simulink model "Vorlage_Anlagenteil_Pruefen_Gruppen12"  (R2023a)
settings: Solver=ode3  StartTime=0.0  StopTime=50  FixedStep=0.01  RelTol=1e-3
StopFcn:
  | clear con
model workspace (MAT data in the model file):
  A = Simulink.Signal
  A.DataType = 'auto'
  A.Dimensions = 1
  A.DimensionsMode = 'auto'
  A.Complexity = 'auto'
  A.SampleTime = -1
  A.SamplingMode = 'auto'
undefined symbols (not defined in the file): sigbuilder_block
libraries: simulink x11, simulink_extras x6, aerolibanimutils x1
(part 1 of 2)
settings Model: Creator=Jan  LastModifiedBy=ASUS
settings SolverCC: AlgebraicLoopSolver=TrustRegion
settings DataIOCC: ReturnWorkspaceOutputs=off
settings DebuggingCC: UnconnectedInputMsg=warning  UnconnectedOutputMsg=warning  UnconnectedLineMsg=warning  ArithmeticOperatorsInVariantConditions=warning
settings ModelReferenceCC: EnableRefExpFcnMdlSchedulingChecks=on
settings SFSimCC: SimUseLocalCustomCode=off  CustomCodeUndefinedFunction=UseInterfaceOnly
settings RTWCC: RTWUseLocalCustomCode=off  DLArmComputeVersion=19.05
settings CodeAppCC: StateflowObjectComments=on
settings SimscapeCC: SimscapeNormalizeSystem=off

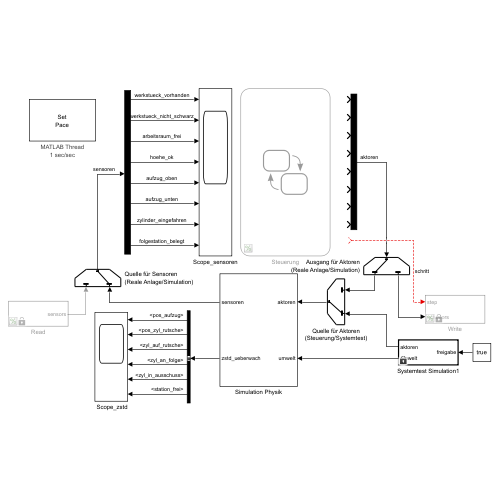
[thumbnail: Simulink's stored preview of the top-level diagram]
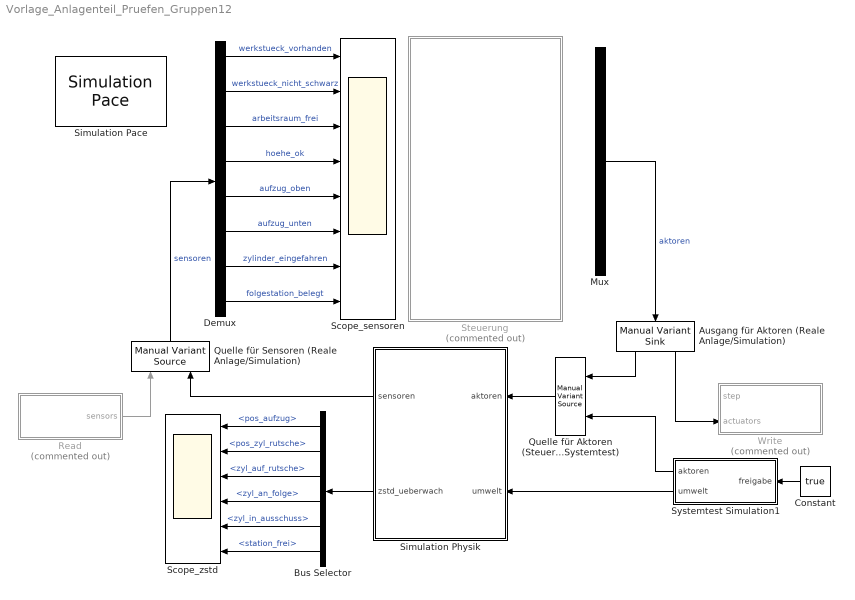
== system Vorlage_Anlagenteil_Pruefen_Gruppen12 ==
  " Scope_zstd" : Scope  NumInputPorts=6
  Ausgang für Aktoren (Reale Anlage/Simulation) : simulink/Signal Routing/Manual Variant Sink  NumChoices=2  LabelModeActiveChoice=V_1
  Bus Selector : BusSelector  OutputSignals=pos_aufzug,pos_zyl_rutsche,zyl_auf_rutsche,zyl_an_folge,zyl_in_ausschuss,station_frei
  Constant : Constant  Value=true
  Demux : Demux  Outputs=8
  Mux : Mux  Inputs=8
  Quelle für Aktoren (Steuerung/Systemtest) : simulink/Signal Routing/Manual Variant Source  NumChoices=2  LabelModeActiveChoice=V_2
  Quelle für Sensoren (Reale Anlage/Simulation) : simulink/Signal Routing/Manual Variant Source  NumChoices=2  LabelModeActiveChoice=V_2
  Read : Subsystem  Commented=on
  Scope_sensoren : Scope  NumInputPorts=8
  Simulation Pace : aerolibanimutils/Simulation Pace  SimulationPace=1  SleepMode=MATLAB Thread  OutputPaceError=off  SampleTime=-1
  Simulation Physik : Subsystem
  Steuerung : Stateflow chart  Commented=on  TreatAsAtomicUnit=on
  Systemtest Simulation1 : Subsystem  TreatAsAtomicUnit=on
  Write : Subsystem  Commented=on
  wires:
  Quelle für Sensoren (Reale Anlage/Simulation)/1 -> Demux/1  "sensoren"
  Read/1(sensors) -> Quelle für Sensoren (Reale Anlage/Simulation)/1
  Mux/1 -> Ausgang für Aktoren (Reale Anlage/Simulation)/1  "aktoren"
  Simulation Physik/1(sensoren) -> Quelle für Sensoren (Reale Anlage/Simulation)/2
  Ausgang für Aktoren (Reale Anlage/Simulation)/2 -> Write/2(actuators)
  Ausgang für Aktoren (Reale Anlage/Simulation)/1 -> Quelle für Aktoren (Steuerung/Systemtest)/1
  Quelle für Aktoren (Steuerung/Systemtest)/1 -> Simulation Physik/1(aktoren)
  Systemtest Simulation1/1(aktoren) -> Quelle für Aktoren (Steuerung/Systemtest)/2
  Systemtest Simulation1/2(umwelt) -> Simulation Physik/2(umwelt)
  Simulation Physik/2(zstd_ueberwach) -> Bus Selector/1
  Bus Selector/1 -> " Scope_zstd"/1  "<pos_aufzug>"
  Bus Selector/2 -> " Scope_zstd"/2  "<pos_zyl_rutsche>"
  Bus Selector/3 -> " Scope_zstd"/3  "<zyl_auf_rutsche>"
  Bus Selector/4 -> " Scope_zstd"/4  "<zyl_an_folge>"
  Bus Selector/5 -> " Scope_zstd"/5  "<zyl_in_ausschuss>"
  Bus Selector/6 -> " Scope_zstd"/6  "<station_frei>"
  Demux/1 -> Scope_sensoren/1  "werkstueck_vorhanden"
  Demux/2 -> Scope_sensoren/2  "werkstueck_nicht_schwarz"
  Demux/3 -> Scope_sensoren/3  "arbeitsraum_frei"
  Demux/4 -> Scope_sensoren/4  "hoehe_ok"
  Demux/5 -> Scope_sensoren/5  "aufzug_oben"
  Demux/6 -> Scope_sensoren/6  "aufzug_unten"
  Demux/7 -> Scope_sensoren/7  "zylinder_eingefahren"
  Demux/8 -> Scope_sensoren/8  "folgestation_belegt"
  ? -> Write/1(step)  "schritt"
  Constant/1 -> Systemtest Simulation1/1(freigabe)

== system Vorlage_Anlagenteil_Pruefen_Gruppen12/Read ==
  Read : MATLAB Function  TreatAsAtomicUnit=on
  sensors : Outport  VectorParamsAs1DForOutWhenUnconnected=off
  wires:
  Read/1(senarr) -> sensors/1

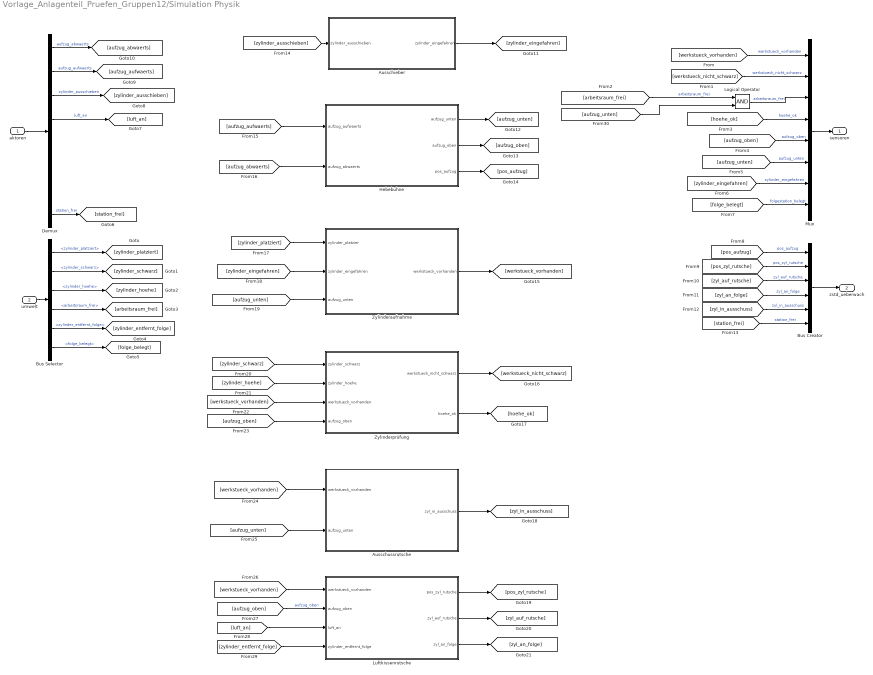
== system Vorlage_Anlagenteil_Pruefen_Gruppen12/Simulation Physik ==
  aktoren : Inport
  umwelt : Inport  Port=2
  Ausschieber : Subsystem
  Ausschussrutsche : Subsystem  TreatAsAtomicUnit=on
  Bus Creator : BusCreator  Inputs=6
  Bus Selector : BusSelector  OutputSignals=zylinder_platziert,zylinder_schwarz,zylinder_hoehe,arbeitsraum_frei,zylinder_entfernt_folge,folge_belegt
  Demux : Demux  Outputs=8
  "Hebebühne " : Subsystem
  Logical Operator : Logic  AllPortsSameDT=off  OutDataTypeStr=boolean
  Luftkissenrutsche : Subsystem
  Mux : Mux  Inputs=8
  Zylinderaufnahme : Subsystem
  Zylinderprüfung : Subsystem
  sensoren : Outport  VectorParamsAs1DForOutWhenUnconnected=off
  zstd_ueberwach : Outport  Port=2  VectorParamsAs1DForOutWhenUnconnected=off
  wires:
  aktoren/1 -> Demux/1
  Mux/1 -> sensoren/1
  Demux/1 -> [aufzug_abwaerts]  "aufzug_abwaerts"
  [folge_belegt] -> Mux/8  "folgestation_belegt"
  Demux/2 -> [aufzug_aufwaerts]  "aufzug_aufwaerts"
  Demux/3 -> [zylinder_ausschieben]  "zylinder_ausschieben"
  [werkstueck_vorhanden] -> Mux/1  "werkstueck_vorhanden"
  [hoehe_ok] -> Mux/4  "hoehe_ok"
  [werkstueck_nicht_schwarz] -> Mux/2  "werkstueck_nicht_schwarz"
  umwelt/1 -> Bus Selector/1
  Bus Selector/1 -> [zylinder_platziert]  "<zylinder_platziert>"
  Bus Selector/2 -> [zylinder_schwarz]  "<zylinder_schwarz>"
  Bus Selector/4 -> [arbeitsraum_frei]  "<arbeitsraum_frei>"
  Bus Selector/5 -> [zylinder_entfernt_folge]  "<zylinder_entfernt_folge>"
  Bus Selector/6 -> [folge_belegt]  "<folge_belegt>"
  [pos_aufzug] -> Bus Creator/1  "pos_aufzug"
  Bus Creator/1 -> zstd_ueberwach/1
  [pos_zyl_rutsche] -> Bus Creator/2  "pos_zyl_rutsche"
  [zyl_auf_rutsche] -> Bus Creator/3  "zyl_auf_rutsche"
  [zyl_an_folge] -> Bus Creator/4  "zyl_an_folge"
  [zyl_in_ausschuss] -> Bus Creator/5  "zyl_in_ausschuss"
  [aufzug_unten] -> Mux/6  "aufzug_unten"
  [zylinder_eingefahren] -> Mux/7  "zylinder_eingefahren"
  [aufzug_oben] -> Mux/5  "aufzug_oben"
  Bus Selector/3 -> [zylinder_hoehe]  "<zylinder_hoehe>"
  Demux/8 -> [station_frei]  "station_frei"
  [station_frei] -> Bus Creator/6  "station_frei"
  Demux/4 -> [luft_an]  "luft_an"
  [zylinder_ausschieben] -> Ausschieber/1(zylinder_ausschieben)
  Ausschieber/1(zylinder_eingefahren) -> [zylinder_eingefahren]
  [aufzug_aufwaerts] -> "Hebebühne "/1(aufzug_aufwaerts)
  [aufzug_abwaerts] -> "Hebebühne "/2(aufzug_abwaerts)
  "Hebebühne "/1(aufzug_unten) -> [aufzug_unten]
  "Hebebühne "/2(aufzug_oben) -> [aufzug_oben]
  "Hebebühne "/3(pos_aufzug) -> [pos_aufzug]
  [aufzug_unten] -> Zylinderaufnahme/3(aufzug_unten)
  [zylinder_eingefahren] -> Zylinderaufnahme/2(zylinder_eingefahren)
  [zylinder_platziert] -> Zylinderaufnahme/1(zylinder_platzier)
  Zylinderaufnahme/1(werkstueck_vorhanden) -> [werkstueck_vorhanden]
  [zylinder_schwarz] -> Zylinderprüfung/1(zylinder_schwarz)
  [zylinder_hoehe] -> Zylinderprüfung/2(zylinder_hoehe)
  [werkstueck_vorhanden] -> Zylinderprüfung/3(werkstueck_vorhanden)
  [aufzug_oben] -> Zylinderprüfung/4("aufzug_oben ")
  Zylinderprüfung/1(werkstueck_nicht_schwarz) -> [werkstueck_nicht_schwarz]
  Zylinderprüfung/2(hoehe_ok) -> [hoehe_ok]
  [aufzug_unten] -> Ausschussrutsche/2("aufzug_unten ")
  [werkstueck_vorhanden] -> Ausschussrutsche/1(werkstueck_vorhanden)
  Ausschussrutsche/1(zyl_in_ausschuss) -> [zyl_in_ausschuss]
  Luftkissenrutsche/1(pos_zyl_rutsche) -> [pos_zyl_rutsche]
  Luftkissenrutsche/3(zyl_an_folge) -> [zyl_an_folge]
  Luftkissenrutsche/2(zyl_auf_rutsche) -> [zyl_auf_rutsche]
  [werkstueck_vorhanden] -> Luftkissenrutsche/1("werkstueck_vorhanden ")
  [aufzug_oben] -> Luftkissenrutsche/2("aufzug_oben ")  "aufzug_oben"
  [luft_an] -> Luftkissenrutsche/3(luft_an)
  [zylinder_entfernt_folge] -> Luftkissenrutsche/4(zylinder_entfernt_folge)
  [arbeitsraum_frei] -> Logical Operator/1  "arbeitsraum_frei"
  Logical Operator/1 -> Mux/3  "arbeitsraum_frei"
  [aufzug_unten] -> Logical Operator/2

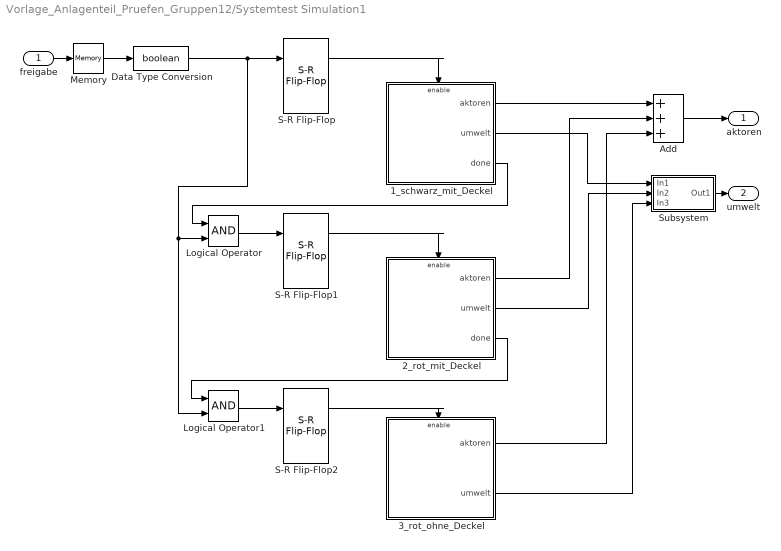
== system Vorlage_Anlagenteil_Pruefen_Gruppen12/Systemtest Simulation1 ==
  freigabe : Inport
  1_schwarz_mit_Deckel : Subsystem
  2_rot_mit_Deckel : Subsystem
  3_rot_ohne_Deckel : Subsystem
  Add : Sum  Inputs=+++
  Data Type Conversion : DataTypeConversion  OutDataTypeStr=boolean  SaturateOnIntegerOverflow=off  RndMeth=Floor
  Logical Operator : Logic  AllPortsSameDT=off  OutDataTypeStr=boolean
  Logical Operator1 : Logic  AllPortsSameDT=off  OutDataTypeStr=boolean
  Memory : Memory
  S-R Flip-Flop : simulink_extras/Flip Flops/S-R Flip-Flop  initial_condition=0
  S-R Flip-Flop1 : simulink_extras/Flip Flops/S-R Flip-Flop  initial_condition=0
  S-R Flip-Flop2 : simulink_extras/Flip Flops/S-R Flip-Flop  initial_condition=0
  Subsystem : Subsystem
  aktoren : Outport  VectorParamsAs1DForOutWhenUnconnected=off
  umwelt : Outport  Port=2  VectorParamsAs1DForOutWhenUnconnected=off
  wires:
  freigabe/1 -> Memory/1
  S-R Flip-Flop/1 -> 1_schwarz_mit_Deckel/Enable
  Logical Operator/1 -> S-R Flip-Flop1/1
  1_schwarz_mit_Deckel/3(done) -> Logical Operator/1
  S-R Flip-Flop1/1 -> 2_rot_mit_Deckel/Enable
  Logical Operator1/1 -> S-R Flip-Flop2/1
  2_rot_mit_Deckel/3(done) -> Logical Operator1/1
  S-R Flip-Flop2/1 -> 3_rot_ohne_Deckel/Enable
  1_schwarz_mit_Deckel/1(aktoren) -> Add/1
  2_rot_mit_Deckel/1(aktoren) -> Add/2
  Add/1 -> aktoren/1
  3_rot_ohne_Deckel/1(aktoren) -> Add/3
  Subsystem/1(Out1) -> umwelt/1
  1_schwarz_mit_Deckel/2(umwelt) -> Subsystem/1(In1)
  2_rot_mit_Deckel/2(umwelt) -> Subsystem/2(In2)
  3_rot_ohne_Deckel/2(umwelt) -> Subsystem/3(In3)
  Data Type Conversion/1 -> Logical Operator1/2, Logical Operator/2, S-R Flip-Flop/1
  Memory/1 -> Data Type Conversion/1

== system Vorlage_Anlagenteil_Pruefen_Gruppen12/Write ==
  step : Inport
  actuators : Inport  Port=2
  Data Type Conversion : DataTypeConversion  OutDataTypeStr=boolean  SaturateOnIntegerOverflow=off  RndMeth=Floor
  Write1 : MATLAB Function  TreatAsAtomicUnit=on
  wires:
  step/1 -> Write1/1(step)
  Data Type Conversion/1 -> Write1/2(actuators)
  actuators/1 -> Data Type Conversion/1

== system Vorlage_Anlagenteil_Pruefen_Gruppen12/Simulation Physik/Ausschieber ==
  zylinder_ausschieben : Inport
  " " : Logic  Operator=NOT  AllPortsSameDT=off  OutDataTypeStr=boolean
  "  " : Delay  DelayLength=50
  Scope : Scope  NumInputPorts=2
  zylinder_eingefahren : Outport
  wires:
  zylinder_ausschieben/1 -> Scope/2, " "/1  "zylinder_ausschieben"
  " "/1 -> "  "/1
  "  "/1 -> Scope/1, zylinder_eingefahren/1  "zylinder_eingefahren"

== system Vorlage_Anlagenteil_Pruefen_Gruppen12/Simulation Physik/Ausschussrutsche ==
  werkstueck_vorhanden : Inport
  "aufzug_unten " : Inport  Port=2
  AND : Logic  IconShape=distinctive  AllPortsSameDT=off  OutDataTypeStr=boolean
  Detect Fall Nonpositive : simulink/Logic and Bit Operations/Detect Fall Nonpositive  vinit=0  OutDataTypeStr=boolean
  Scope : Scope  NumInputPorts=3
  Triggered Subsystem : Subsystem  TreatAsAtomicUnit=on
  zyl_in_ausschuss : Outport
  wires:
  werkstueck_vorhanden/1 -> Scope/1, Detect Fall Nonpositive/1  "werkstueck_vorhanden"
  Detect Fall Nonpositive/1 -> AND/1
  "aufzug_unten "/1 -> Scope/2, AND/2  "aufzug_unten"
  AND/1 -> Triggered Subsystem/Trigger
  Triggered Subsystem/1(zyl_in_ausschuss) -> Scope/3, zyl_in_ausschuss/1  "zyl_in_ausschuss"

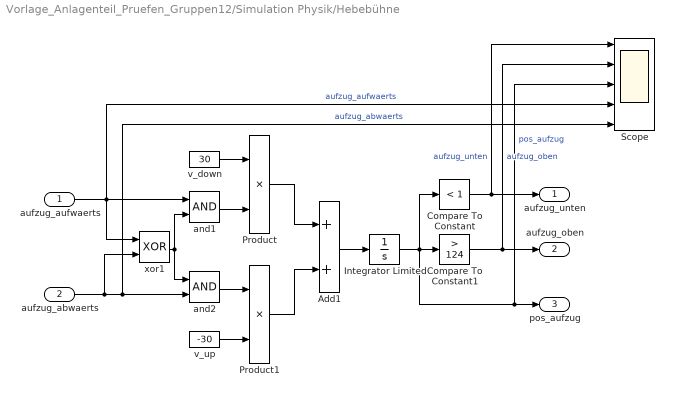
== system Vorlage_Anlagenteil_Pruefen_Gruppen12/Simulation Physik/Hebebühne  ==
  aufzug_aufwaerts : Inport
  aufzug_abwaerts : Inport  Port=2
  Add1 : Sum
  Compare To Constant : simulink/Logic and Bit Operations/Compare To Constant  relop=<  const=1  OutDataTypeStr=boolean
  Compare To Constant1 : simulink/Logic and Bit Operations/Compare To Constant  relop=>  const=124  OutDataTypeStr=boolean
  Integrator Limited : Integrator  LimitOutput=on  UpperSaturationLimit=125  LowerSaturationLimit=0
  Product : Product
  Product1 : Product
  Scope : Scope  NumInputPorts=5
  and1 : Logic  AllPortsSameDT=off  OutDataTypeStr=boolean
  and2 : Logic  AllPortsSameDT=off  OutDataTypeStr=boolean
  v_down : Constant  Value=30
  v_up : Constant  Value=-30
  xor1 : Logic  Operator=XOR  AllPortsSameDT=off  OutDataTypeStr=boolean
  aufzug_unten : Outport
  aufzug_oben : Outport  Port=2
  pos_aufzug : Outport  Port=3
  wires:
  Compare To Constant/1 -> Scope/1, aufzug_unten/1  "aufzug_unten"
  Integrator Limited/1 -> pos_aufzug/1, Scope/3, Compare To Constant/1, Compare To Constant1/1  "pos_aufzug"
  Add1/1 -> Integrator Limited/1
  Product1/1 -> Add1/2
  Product/1 -> Add1/1
  v_up/1 -> Product1/2
  and2/1 -> Product1/1
  v_down/1 -> Product/1
  and1/1 -> Product/2
  xor1/1 -> and1/2, and2/1
  aufzug_aufwaerts/1 -> Scope/4, and1/1, xor1/1  "aufzug_aufwaerts"
  aufzug_abwaerts/1 -> Scope/5, and2/2, xor1/2  "aufzug_abwaerts"
  Compare To Constant1/1 -> aufzug_oben/1, Scope/2  "aufzug_oben"

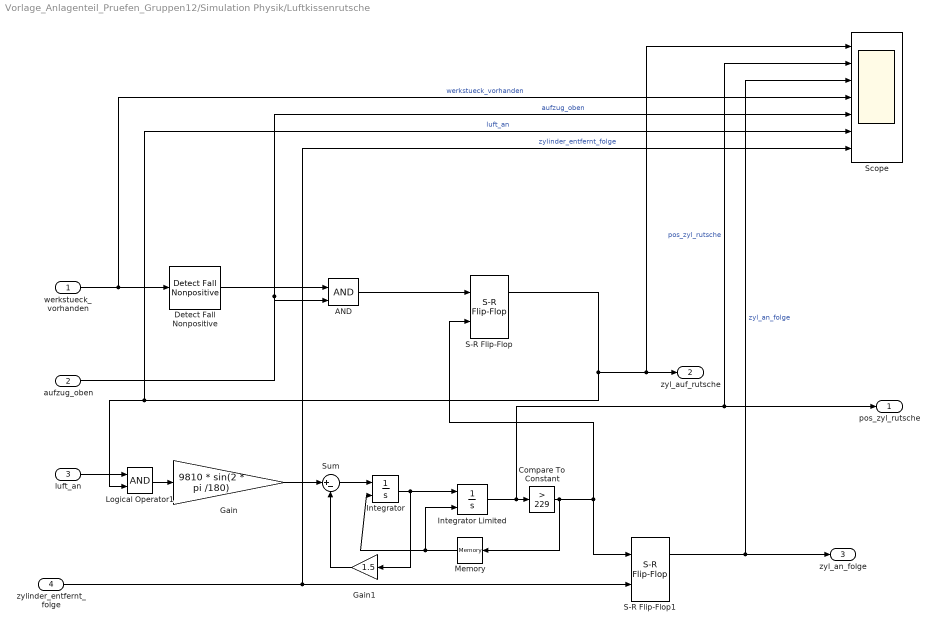
== system Vorlage_Anlagenteil_Pruefen_Gruppen12/Simulation Physik/Luftkissenrutsche ==
  "werkstueck_vorhanden " : Inport
  "aufzug_oben " : Inport  Port=2
  luft_an : Inport  Port=3
  zylinder_entfernt_folge : Inport  Port=4
  AND : Logic  IconShape=distinctive  AllPortsSameDT=off  OutDataTypeStr=boolean
  Compare To Constant : simulink/Logic and Bit Operations/Compare To Constant  relop=>  const=229  OutDataTypeStr=boolean
  Detect Fall Nonpositive : simulink/Logic and Bit Operations/Detect Fall Nonpositive  vinit=0  OutDataTypeStr=boolean
  Gain : Gain  Gain=9810 * sin(2 * pi /180)
  Gain1 : Gain  Gain=1.5
  Integrator : Integrator  ExternalReset=rising
  Integrator Limited : Integrator  ExternalReset=rising  LimitOutput=on  UpperSaturationLimit=230  LowerSaturationLimit=0
  Logical Operator1 : Logic  AllPortsSameDT=off  OutDataTypeStr=boolean
  Memory : Memory
  S-R Flip-Flop : simulink_extras/Flip Flops/S-R Flip-Flop  initial_condition=0
  S-R Flip-Flop1 : simulink_extras/Flip Flops/S-R Flip-Flop  initial_condition=0
  Scope : Scope  NumInputPorts=7
  Sum : Sum  Inputs=|+-
  pos_zyl_rutsche : Outport
  zyl_auf_rutsche : Outport  Port=2
  zyl_an_folge : Outport  Port=3
  wires:
  "werkstueck_vorhanden "/1 -> Scope/4, Detect Fall Nonpositive/1  "werkstueck_vorhanden"
  Detect Fall Nonpositive/1 -> AND/1
  "aufzug_oben "/1 -> Scope/5, AND/2  "aufzug_oben"
  zylinder_entfernt_folge/1 -> Scope/7, S-R Flip-Flop1/2  "zylinder_entfernt_folge"
  S-R Flip-Flop1/1 -> Scope/3, zyl_an_folge/1  "zyl_an_folge"
  Gain1/1 -> Sum/2
  Memory/1 -> Integrator/2, Integrator Limited/2
  Compare To Constant/1 -> S-R Flip-Flop/2, S-R Flip-Flop1/1, Memory/1
  Integrator Limited/1 -> pos_zyl_rutsche/1, Scope/2, Compare To Constant/1  "pos_zyl_rutsche"
  Integrator/1 -> Integrator Limited/1, Gain1/1
  Sum/1 -> Integrator/1
  Gain/1 -> Sum/1
  Logical Operator1/1 -> Gain/1
  luft_an/1 -> Logical Operator1/1
  S-R Flip-Flop/1 -> Scope/1, zyl_auf_rutsche/1, Logical Operator1/2, Scope/6  "luft_an"
  AND/1 -> S-R Flip-Flop/1

== system Vorlage_Anlagenteil_Pruefen_Gruppen12/Simulation Physik/Zylinderaufnahme ==
  zylinder_platzier : Inport
  zylinder_eingefahren : Inport  Port=2
  aufzug_unten : Inport  Port=3
  Detect Fall Nonpositive : simulink/Logic and Bit Operations/Detect Fall Nonpositive  vinit=0  OutDataTypeStr=boolean
  Detect Rise Positive : simulink/Logic and Bit Operations/Detect Rise Positive  vinit=0  OutDataTypeStr=boolean
  Logical Operator : Logic  Inputs=3  AllPortsSameDT=off  OutDataTypeStr=boolean
  S-R Flip-Flop : simulink_extras/Flip Flops/S-R Flip-Flop  initial_condition=0
  Scope : Scope  NumInputPorts=4
  werkstueck_vorhanden : Outport
  wires:
  zylinder_platzier/1 -> Scope/2, Detect Rise Positive/1  "zylinder_platzier"
  Detect Rise Positive/1 -> Logical Operator/1
  aufzug_unten/1 -> Scope/4, Logical Operator/3  "aufzug_unten"
  zylinder_eingefahren/1 -> Scope/3, Logical Operator/2, Detect Fall Nonpositive/1  "zylinder_eingefahren"
  Detect Fall Nonpositive/1 -> S-R Flip-Flop/2
  Logical Operator/1 -> S-R Flip-Flop/1
  S-R Flip-Flop/1 -> Scope/1, werkstueck_vorhanden/1  "werkstueck_vorhanden"

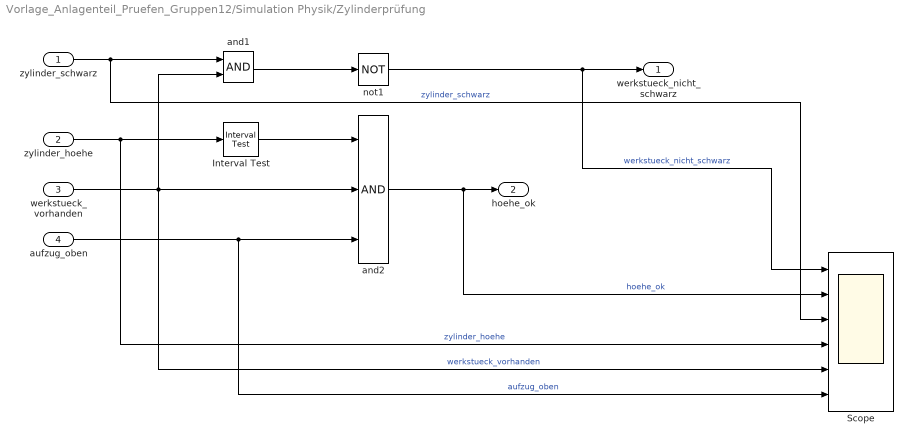
== system Vorlage_Anlagenteil_Pruefen_Gruppen12/Simulation Physik/Zylinderprüfung ==
  zylinder_schwarz : Inport
  zylinder_hoehe : Inport  Port=2
  werkstueck_vorhanden : Inport  Port=3
  "aufzug_oben " : Inport  Port=4
  Interval Test : simulink/Logic and Bit Operations/Interval Test  IntervalClosedRight=on  uplimit=26  IntervalClosedLeft=on  lowlimit=24  OutDataTypeStr=boolean
  Scope : Scope  NumInputPorts=6
  and1 : Logic  AllPortsSameDT=off  OutDataTypeStr=boolean
  and2 : Logic  Inputs=3  AllPortsSameDT=off  OutDataTypeStr=boolean
  not1 : Logic  Operator=NOT  AllPortsSameDT=off  OutDataTypeStr=boolean
  werkstueck_nicht_schwarz : Outport
  hoehe_ok : Outport  Port=2
  wires:
  zylinder_schwarz/1 -> Scope/3, and1/1  "zylinder_schwarz"
  werkstueck_vorhanden/1 -> Scope/5, and1/2, and2/2  "werkstueck_vorhanden"
  and1/1 -> not1/1
  not1/1 -> Scope/1, werkstueck_nicht_schwarz/1  "werkstueck_nicht_schwarz"
  zylinder_hoehe/1 -> Scope/4, Interval Test/1  "zylinder_hoehe"
  and2/1 -> Scope/2, hoehe_ok/1  "hoehe_ok"
  Interval Test/1 -> and2/1
  "aufzug_oben "/1 -> Scope/6, and2/3  "aufzug_oben"

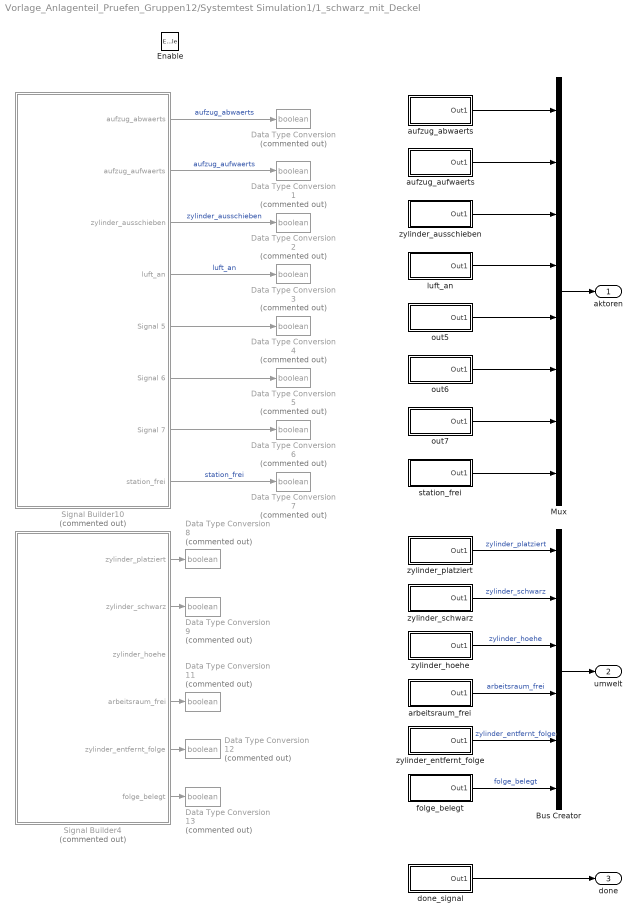
== system Vorlage_Anlagenteil_Pruefen_Gruppen12/Systemtest Simulation1/1_schwarz_mit_Deckel ==
  Enable : EnablePort
  Bus Creator : BusCreator  Inputs=6
  Data Type Conversion{,1..9,11..13} (13 alike) : DataTypeConversion  Commented=on  OutDataTypeStr=boolean  SaturateOnIntegerOverflow=off  RndMeth=Floor
  Mux : Mux  Inputs=8
  Signal Builder10 : Subsystem  Tag=STV Subsys  Commented=on  LoadFcn=sigbuilder_block('load');  StartFcn=sigbuilder_block('start');  StopFcn=sigbuilder_block('stop');  ClipboardFcn=sigbuilder_block('clipboard');  mask(Sigbuilder block){tuvar=[0:10]}
      mask help: Simulink:masks:SigbuilderBlock_MD
      mask init:
      | if ~strcmp(get_param(bdroot(gcbh),'SimulationStatus'),'stopped') tuvar = sigbuilder_block('maskInit'); end
      settings: CopyFcn=sigbuilder_block('copy');  DeleteFcn=sigbuilder_block('delete');  ModelCloseFcn=sigbuilder_block('modelClose');  PreSaveFcn=sigbuilder_block('preSave');  PauseFcn=sigbuilder_block('pause');  ContinueFcn=sigbuilder_block('continue');  NameChangeFcn=sigbuilder_block('namechange');  OpenFcn=sigbuilder_block('open',[2160 -195 1440 817.5 ]);  CloseFcn=sigbuilder_block('close');
      mask Display: plot(0, 0, 100, 100,[2, 2, 32, 32, 2], [68, 8, 8, 68, 68],[32, 2], [38, 38], [32, 19, 2],[53, 60, 44], [32, 17, 17, 2],[16, 16, 31, 31]);txt = getActiveGroup(gcbh);text(2, 100, txt,'verticalAlignment', 'top');
  Signal Builder4 : Subsystem  Tag=STV Subsys  Commented=on  LoadFcn=sigbuilder_block('load');  StartFcn=sigbuilder_block('start');  StopFcn=sigbuilder_block('stop');  ClipboardFcn=sigbuilder_block('clipboard');  mask(Sigbuilder block){tuvar=[0:10]}
      mask help: Simulink:masks:SigbuilderBlock_MD
      mask init:
      | if ~strcmp(get_param(bdroot(gcbh),'SimulationStatus'),'stopped') tuvar = sigbuilder_block('maskInit'); end
      settings: CopyFcn=sigbuilder_block('copy');  DeleteFcn=sigbuilder_block('delete');  ModelCloseFcn=sigbuilder_block('modelClose');  PreSaveFcn=sigbuilder_block('preSave');  PauseFcn=sigbuilder_block('pause');  ContinueFcn=sigbuilder_block('continue');  NameChangeFcn=sigbuilder_block('namechange');  OpenFcn=sigbuilder_block('open',[4.875 4.875 1070.25 612.75 ]);  CloseFcn=sigbuilder_block('close');
      mask Display: plot(0, 0, 100, 100,[2, 2, 32, 32, 2], [68, 8, 8, 68, 68],[32, 2], [38, 38], [32, 19, 2],[53, 60, 44], [32, 17, 17, 2],[16, 16, 31, 31]);txt = getActiveGroup(gcbh);text(2, 100, txt,'verticalAlignment', 'top');
  arbeitsraum_frei : Subsystem
  aufzug_abwaerts : Subsystem
  aufzug_aufwaerts : Subsystem
  done_signal : Subsystem
  folge_belegt : Subsystem
  luft_an : Subsystem
  out5 : Subsystem
  out6 : Subsystem
  out7 : Subsystem
  station_frei : Subsystem
  zylinder_ausschieben : Subsystem
  zylinder_entfernt_folge : Subsystem
  zylinder_hoehe : Subsystem
  zylinder_platziert : Subsystem
  zylinder_schwarz : Subsystem
  aktoren : Outport  VectorParamsAs1DForOutWhenUnconnected=off
  umwelt : Outport  Port=2  VectorParamsAs1DForOutWhenUnconnected=off
  done : Outport  Port=3  VectorParamsAs1DForOutWhenUnconnected=off
  wires:
  Bus Creator/1 -> umwelt/1
  Signal Builder4/1(zylinder_platziert) -> Data Type Conversion8/1
  Signal Builder4/2(zylinder_schwarz) -> Data Type Conversion9/1
  zylinder_hoehe/1(Out1) -> Bus Creator/3  "zylinder_hoehe"
  Signal Builder4/4(arbeitsraum_frei) -> Data Type Conversion11/1
  Signal Builder4/5(zylinder_entfernt_folge) -> Data Type Conversion12/1
  Signal Builder4/6(folge_belegt) -> Data Type Conversion13/1
  zylinder_platziert/1(Out1) -> Bus Creator/1  "zylinder_platziert"
  zylinder_schwarz/1(Out1) -> Bus Creator/2  "zylinder_schwarz"
  arbeitsraum_frei/1(Out1) -> Bus Creator/4  "arbeitsraum_frei"
  zylinder_entfernt_folge/1(Out1) -> Bus Creator/5  "zylinder_entfernt_folge"
  folge_belegt/1(Out1) -> Bus Creator/6  "folge_belegt"
  Mux/1 -> aktoren/1
  Signal Builder10/1(aufzug_abwaerts) -> Data Type Conversion/1  "aufzug_abwaerts"
  Signal Builder10/2(aufzug_aufwaerts) -> Data Type Conversion1/1  "aufzug_aufwaerts"
  Signal Builder10/3(zylinder_ausschieben) -> Data Type Conversion2/1  "zylinder_ausschieben"
  Signal Builder10/4(luft_an) -> Data Type Conversion3/1  "luft_an"
  Signal Builder10/8(station_frei) -> Data Type Conversion7/1  "station_frei"
  Signal Builder10/5(Signal 5) -> Data Type Conversion4/1
  Signal Builder10/6(Signal 6) -> Data Type Conversion5/1
  Signal Builder10/7(Signal 7) -> Data Type Conversion6/1
  aufzug_abwaerts/1(Out1) -> Mux/1
  aufzug_aufwaerts/1(Out1) -> Mux/2
  zylinder_ausschieben/1(Out1) -> Mux/3
  luft_an/1(Out1) -> Mux/4
  out5/1(Out1) -> Mux/5
  out6/1(Out1) -> Mux/6
  out7/1(Out1) -> Mux/7
  station_frei/1(Out1) -> Mux/8
  done_signal/1(Out1) -> done/1

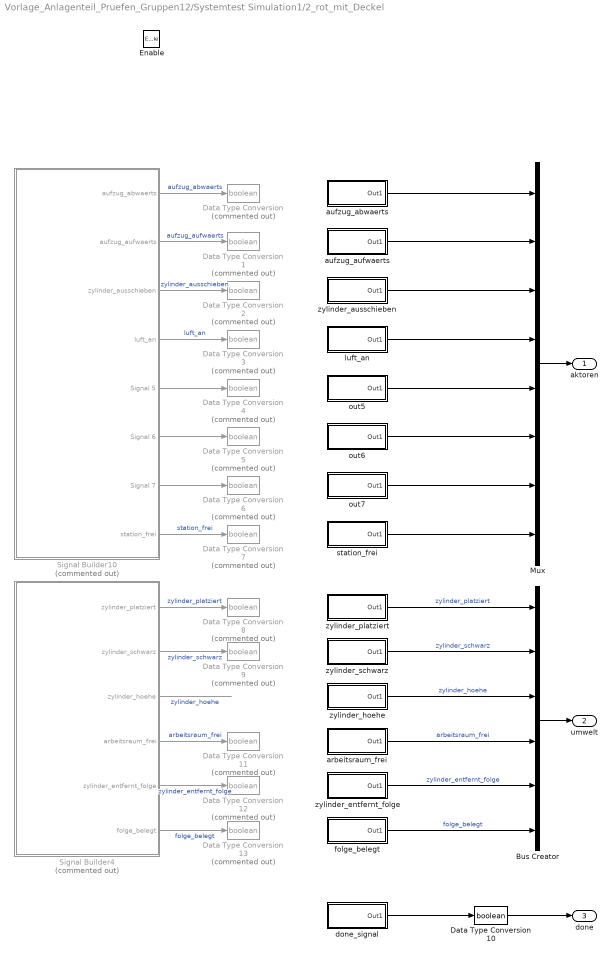
== system Vorlage_Anlagenteil_Pruefen_Gruppen12/Systemtest Simulation1/2_rot_mit_Deckel ==
  Enable : EnablePort
  Bus Creator : BusCreator  Inputs=6
  Data Type Conversion{,1..9,11..13} (13 alike) : DataTypeConversion  Commented=on  OutDataTypeStr=boolean  SaturateOnIntegerOverflow=off  RndMeth=Floor
  Data Type Conversion10 : DataTypeConversion  OutDataTypeStr=boolean  SaturateOnIntegerOverflow=off  RndMeth=Floor
  Mux : Mux  Inputs=8
  Signal Builder10 : Subsystem  Tag=STV Subsys  Commented=on  LoadFcn=sigbuilder_block('load');  StartFcn=sigbuilder_block('start');  StopFcn=sigbuilder_block('stop');  ClipboardFcn=sigbuilder_block('clipboard');  mask(Sigbuilder block){tuvar=[0:10]}
      mask help: Simulink:masks:SigbuilderBlock_MD
      mask init:
      | if ~strcmp(get_param(bdroot(gcbh),'SimulationStatus'),'stopped') tuvar = sigbuilder_block('maskInit'); end
      settings: CopyFcn=sigbuilder_block('copy');  DeleteFcn=sigbuilder_block('delete');  ModelCloseFcn=sigbuilder_block('modelClose');  PreSaveFcn=sigbuilder_block('preSave');  PauseFcn=sigbuilder_block('pause');  ContinueFcn=sigbuilder_block('continue');  NameChangeFcn=sigbuilder_block('namechange');  OpenFcn=sigbuilder_block('open',[4.875 4.875 1070.25 612.75 ]);  CloseFcn=sigbuilder_block('close');
      mask Display: plot(0, 0, 100, 100,[2, 2, 32, 32, 2], [68, 8, 8, 68, 68],[32, 2], [38, 38], [32, 19, 2],[53, 60, 44], [32, 17, 17, 2],[16, 16, 31, 31]);txt = getActiveGroup(gcbh);text(2, 100, txt,'verticalAlignment', 'top');
  Signal Builder4 : Subsystem  Tag=STV Subsys  Commented=on  LoadFcn=sigbuilder_block('load');  StartFcn=sigbuilder_block('start');  StopFcn=sigbuilder_block('stop');  ClipboardFcn=sigbuilder_block('clipboard');  mask(Sigbuilder block){tuvar=[0:10]}
      mask help: Simulink:masks:SigbuilderBlock_MD
      mask init:
      | if ~strcmp(get_param(bdroot(gcbh),'SimulationStatus'),'stopped') tuvar = sigbuilder_block('maskInit'); end
      settings: CopyFcn=sigbuilder_block('copy');  DeleteFcn=sigbuilder_block('delete');  ModelCloseFcn=sigbuilder_block('modelClose');  PreSaveFcn=sigbuilder_block('preSave');  PauseFcn=sigbuilder_block('pause');  ContinueFcn=sigbuilder_block('continue');  NameChangeFcn=sigbuilder_block('namechange');  OpenFcn=sigbuilder_block('open',[2160 -195 1440 817.5 ]);  CloseFcn=sigbuilder_block('close');
      mask Display: plot(0, 0, 100, 100,[2, 2, 32, 32, 2], [68, 8, 8, 68, 68],[32, 2], [38, 38], [32, 19, 2],[53, 60, 44], [32, 17, 17, 2],[16, 16, 31, 31]);txt = getActiveGroup(gcbh);text(2, 100, txt,'verticalAlignment', 'top');
  arbeitsraum_frei : Subsystem
  aufzug_abwaerts : Subsystem
  aufzug_aufwaerts : Subsystem
  done_signal : Subsystem
  folge_belegt : Subsystem
  luft_an : Subsystem
  out5 : Subsystem
  out6 : Subsystem
  out7 : Subsystem
  station_frei : Subsystem
  zylinder_ausschieben : Subsystem
  zylinder_entfernt_folge : Subsystem
  zylinder_hoehe : Subsystem
  zylinder_platziert : Subsystem
  zylinder_schwarz : Subsystem
  aktoren : Outport  VectorParamsAs1DForOutWhenUnconnected=off
  umwelt : Outport  Port=2  VectorParamsAs1DForOutWhenUnconnected=off
  done : Outport  Port=3  VectorParamsAs1DForOutWhenUnconnected=off
  wires:
  Bus Creator/1 -> umwelt/1
  Signal Builder4/1(zylinder_platziert) -> Data Type Conversion8/1  "zylinder_platziert"
  Signal Builder4/2(zylinder_schwarz) -> Data Type Conversion9/1  "zylinder_schwarz"
  Signal Builder4/3(zylinder_hoehe) -> ?  "zylinder_hoehe"
  Signal Builder4/4(arbeitsraum_frei) -> Data Type Conversion11/1  "arbeitsraum_frei"
  Signal Builder4/5(zylinder_entfernt_folge) -> Data Type Conversion12/1  "zylinder_entfernt_folge"
  Signal Builder4/6(folge_belegt) -> Data Type Conversion13/1  "folge_belegt"
  zylinder_platziert/1(Out1) -> Bus Creator/1  "zylinder_platziert"
  zylinder_schwarz/1(Out1) -> Bus Creator/2  "zylinder_schwarz"
  arbeitsraum_frei/1(Out1) -> Bus Creator/4  "arbeitsraum_frei"
  zylinder_entfernt_folge/1(Out1) -> Bus Creator/5  "zylinder_entfernt_folge"
  folge_belegt/1(Out1) -> Bus Creator/6  "folge_belegt"
  Mux/1 -> aktoren/1
  Signal Builder10/1(aufzug_abwaerts) -> Data Type Conversion/1  "aufzug_abwaerts"
  Signal Builder10/2(aufzug_aufwaerts) -> Data Type Conversion1/1  "aufzug_aufwaerts"
  Signal Builder10/3(zylinder_ausschieben) -> Data Type Conversion2/1  "zylinder_ausschieben"
  Signal Builder10/4(luft_an) -> Data Type Conversion3/1  "luft_an"
  Signal Builder10/8(station_frei) -> Data Type Conversion7/1  "station_frei"
  Signal Builder10/5(Signal 5) -> Data Type Conversion4/1
  Signal Builder10/6(Signal 6) -> Data Type Conversion5/1
  Signal Builder10/7(Signal 7) -> Data Type Conversion6/1
  aufzug_abwaerts/1(Out1) -> Mux/1
  aufzug_aufwaerts/1(Out1) -> Mux/2
  zylinder_ausschieben/1(Out1) -> Mux/3
  luft_an/1(Out1) -> Mux/4
  out5/1(Out1) -> Mux/5
  out6/1(Out1) -> Mux/6
  out7/1(Out1) -> Mux/7
  station_frei/1(Out1) -> Mux/8
  Data Type Conversion10/1 -> done/1
  done_signal/1(Out1) -> Data Type Conversion10/1
  zylinder_hoehe/1(Out1) -> Bus Creator/3  "zylinder_hoehe"

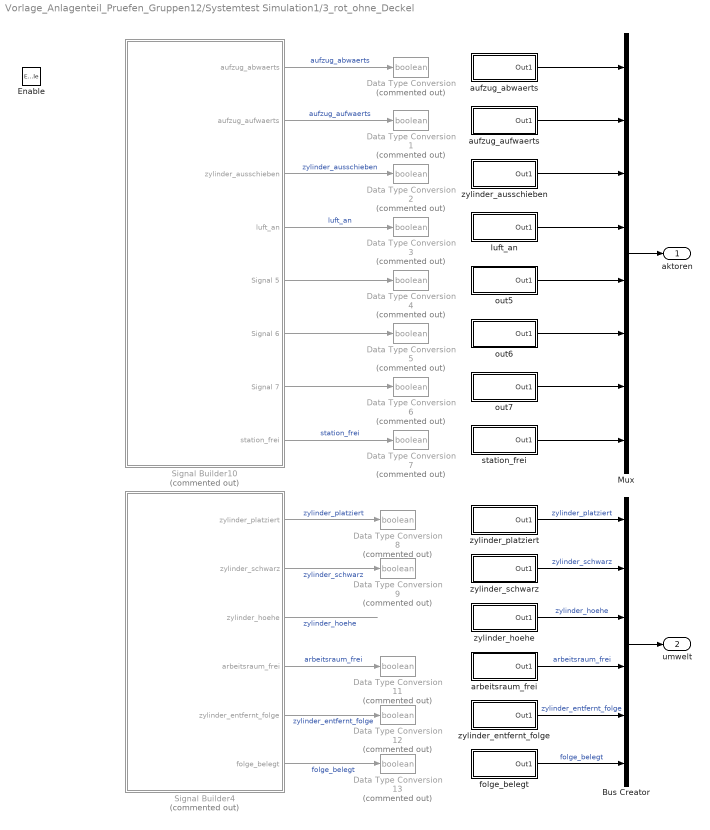
== system Vorlage_Anlagenteil_Pruefen_Gruppen12/Systemtest Simulation1/3_rot_ohne_Deckel ==
  Enable : EnablePort
  Bus Creator : BusCreator  Inputs=6
  Data Type Conversion{,1..9,11..13} (13 alike) : DataTypeConversion  Commented=on  OutDataTypeStr=boolean  SaturateOnIntegerOverflow=off  RndMeth=Floor
  Mux : Mux  Inputs=8
  Signal Builder10 : Subsystem  Tag=STV Subsys  Commented=on  LoadFcn=sigbuilder_block('load');  StartFcn=sigbuilder_block('start');  StopFcn=sigbuilder_block('stop');  ClipboardFcn=sigbuilder_block('clipboard');  mask(Sigbuilder block){tuvar=[0:10]}
      mask help: Simulink:masks:SigbuilderBlock_MD
      mask init:
      | if ~strcmp(get_param(bdroot(gcbh),'SimulationStatus'),'stopped') tuvar = sigbuilder_block('maskInit'); end
      settings: CopyFcn=sigbuilder_block('copy');  DeleteFcn=sigbuilder_block('delete');  ModelCloseFcn=sigbuilder_block('modelClose');  PreSaveFcn=sigbuilder_block('preSave');  PauseFcn=sigbuilder_block('pause');  ContinueFcn=sigbuilder_block('continue');  NameChangeFcn=sigbuilder_block('namechange');  OpenFcn=sigbuilder_block('open',[2160 -195 1440 817.5 ]);  CloseFcn=sigbuilder_block('close');
      mask Display: plot(0, 0, 100, 100,[2, 2, 32, 32, 2], [68, 8, 8, 68, 68],[32, 2], [38, 38], [32, 19, 2],[53, 60, 44], [32, 17, 17, 2],[16, 16, 31, 31]);txt = getActiveGroup(gcbh);text(2, 100, txt,'verticalAlignment', 'top');
  Signal Builder4 : Subsystem  Tag=STV Subsys  Commented=on  LoadFcn=sigbuilder_block('load');  StartFcn=sigbuilder_block('start');  StopFcn=sigbuilder_block('stop');  ClipboardFcn=sigbuilder_block('clipboard');  mask(Sigbuilder block){tuvar=[0:10]}
      mask help: Simulink:masks:SigbuilderBlock_MD
      mask init:
      | if ~strcmp(get_param(bdroot(gcbh),'SimulationStatus'),'stopped') tuvar = sigbuilder_block('maskInit'); end
      settings: CopyFcn=sigbuilder_block('copy');  DeleteFcn=sigbuilder_block('delete');  ModelCloseFcn=sigbuilder_block('modelClose');  PreSaveFcn=sigbuilder_block('preSave');  PauseFcn=sigbuilder_block('pause');  ContinueFcn=sigbuilder_block('continue');  NameChangeFcn=sigbuilder_block('namechange');  OpenFcn=sigbuilder_block('open',[2160 -195 1440 817.5 ]);  CloseFcn=sigbuilder_block('close');
      mask Display: plot(0, 0, 100, 100,[2, 2, 32, 32, 2], [68, 8, 8, 68, 68],[32, 2], [38, 38], [32, 19, 2],[53, 60, 44], [32, 17, 17, 2],[16, 16, 31, 31]);txt = getActiveGroup(gcbh);text(2, 100, txt,'verticalAlignment', 'top');
  arbeitsraum_frei : Subsystem
  aufzug_abwaerts : Subsystem
  aufzug_aufwaerts : Subsystem
  folge_belegt : Subsystem
  luft_an : Subsystem
  out5 : Subsystem
  out6 : Subsystem
  out7 : Subsystem
  station_frei : Subsystem
  zylinder_ausschieben : Subsystem
  zylinder_entfernt_folge : Subsystem
  zylinder_hoehe : Subsystem
  zylinder_platziert : Subsystem
  zylinder_schwarz : Subsystem
  aktoren : Outport  VectorParamsAs1DForOutWhenUnconnected=off
  umwelt : Outport  Port=2  VectorParamsAs1DForOutWhenUnconnected=off
  wires:
  Bus Creator/1 -> umwelt/1
  Signal Builder4/1(zylinder_platziert) -> Data Type Conversion8/1  "zylinder_platziert"
  Signal Builder4/2(zylinder_schwarz) -> Data Type Conversion9/1  "zylinder_schwarz"
  Signal Builder4/3(zylinder_hoehe) -> ?  "zylinder_hoehe"
  Signal Builder4/4(arbeitsraum_frei) -> Data Type Conversion11/1  "arbeitsraum_frei"
  Signal Builder4/5(zylinder_entfernt_folge) -> Data Type Conversion12/1  "zylinder_entfernt_folge"
  Signal Builder4/6(folge_belegt) -> Data Type Conversion13/1  "folge_belegt"
  zylinder_platziert/1(Out1) -> Bus Creator/1  "zylinder_platziert"
  zylinder_schwarz/1(Out1) -> Bus Creator/2  "zylinder_schwarz"
  arbeitsraum_frei/1(Out1) -> Bus Creator/4  "arbeitsraum_frei"
  zylinder_entfernt_folge/1(Out1) -> Bus Creator/5  "zylinder_entfernt_folge"
  folge_belegt/1(Out1) -> Bus Creator/6  "folge_belegt"
  Mux/1 -> aktoren/1
  Signal Builder10/1(aufzug_abwaerts) -> Data Type Conversion/1  "aufzug_abwaerts"
  Signal Builder10/2(aufzug_aufwaerts) -> Data Type Conversion1/1  "aufzug_aufwaerts"
  Signal Builder10/3(zylinder_ausschieben) -> Data Type Conversion2/1  "zylinder_ausschieben"
  Signal Builder10/4(luft_an) -> Data Type Conversion3/1  "luft_an"
  Signal Builder10/8(station_frei) -> Data Type Conversion7/1  "station_frei"
  Signal Builder10/5(Signal 5) -> Data Type Conversion4/1
  Signal Builder10/6(Signal 6) -> Data Type Conversion5/1
  Signal Builder10/7(Signal 7) -> Data Type Conversion6/1
  aufzug_abwaerts/1(Out1) -> Mux/1
  aufzug_aufwaerts/1(Out1) -> Mux/2
  zylinder_ausschieben/1(Out1) -> Mux/3
  luft_an/1(Out1) -> Mux/4
  out5/1(Out1) -> Mux/5
  out6/1(Out1) -> Mux/6
  out7/1(Out1) -> Mux/7
  station_frei/1(Out1) -> Mux/8
  zylinder_hoehe/1(Out1) -> Bus Creator/3  "zylinder_hoehe"

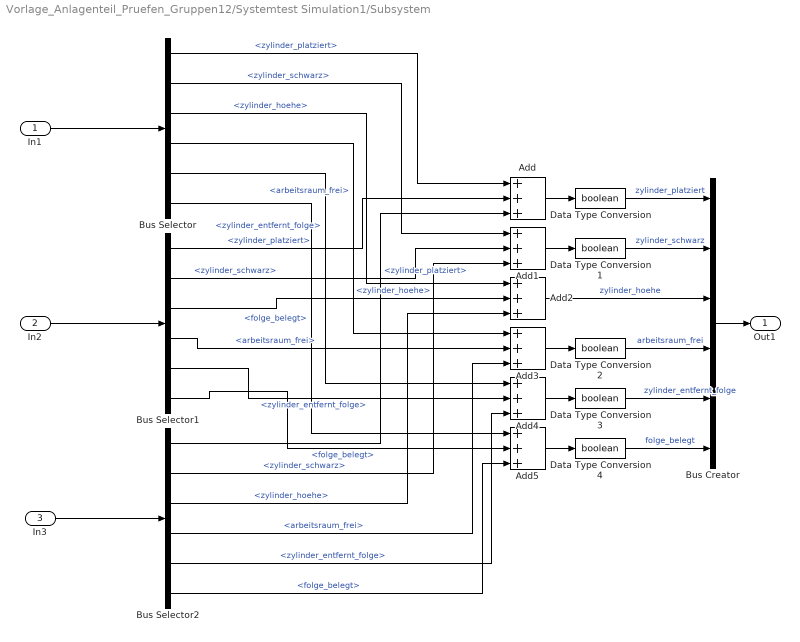
== system Vorlage_Anlagenteil_Pruefen_Gruppen12/Systemtest Simulation1/Subsystem ==
  In1 : Inport
  In2 : Inport  Port=2
  In3 : Inport  Port=3
  Add{,1..5} (6 alike) : Sum  Inputs=+++
  Bus Creator : BusCreator  Inputs=6
  Bus Selector : BusSelector  OutputSignals=zylinder_platziert,zylinder_schwarz,zylinder_hoehe,arbeitsraum_frei,zylinder_entfernt_folge,folge_belegt
  Bus Selector1 : BusSelector  OutputSignals=zylinder_platziert,zylinder_schwarz,zylinder_hoehe,arbeitsraum_frei,zylinder_entfernt_folge,folge_belegt
  Bus Selector2 : BusSelector  OutputSignals=zylinder_platziert,zylinder_schwarz,zylinder_hoehe,arbeitsraum_frei,zylinder_entfernt_folge,folge_belegt
  Data Type Conversion{,1..4} (5 alike) : DataTypeConversion  OutDataTypeStr=boolean  SaturateOnIntegerOverflow=off  RndMeth=Floor
  Out1 : Outport  VectorParamsAs1DForOutWhenUnconnected=off
  wires:
  In1/1 -> Bus Selector/1
  In2/1 -> Bus Selector1/1
  In3/1 -> Bus Selector2/1
  Bus Creator/1 -> Out1/1
  Bus Selector/1 -> Add/1  "<zylinder_platziert>"
  Data Type Conversion/1 -> Bus Creator/1  "zylinder_platziert"
  Bus Selector1/1 -> Add/2  "<zylinder_platziert>"
  Bus Selector2/1 -> Add/3  "<zylinder_platziert>"
  Data Type Conversion1/1 -> Bus Creator/2  "zylinder_schwarz"
  Bus Selector/2 -> Add1/1  "<zylinder_schwarz>"
  Bus Selector1/2 -> Add1/2  "<zylinder_schwarz>"
  Bus Selector2/2 -> Add1/3  "<zylinder_schwarz>"
  Add2/1 -> Bus Creator/3  "zylinder_hoehe"
  Bus Selector/3 -> Add2/1  "<zylinder_hoehe>"
  Bus Selector1/3 -> Add2/2  "<zylinder_hoehe>"
  Bus Selector2/3 -> Add2/3  "<zylinder_hoehe>"
  Add3/1 -> Data Type Conversion2/1
  Bus Selector/4 -> Add3/1  "<arbeitsraum_frei>"
  Bus Selector1/4 -> Add3/2  "<arbeitsraum_frei>"
  Bus Selector2/4 -> Add3/3  "<arbeitsraum_frei>"
  Data Type Conversion3/1 -> Bus Creator/5  "zylinder_entfernt_folge"
  Bus Selector/5 -> Add4/1  "<zylinder_entfernt_folge>"
  Bus Selector1/5 -> Add4/2  "<zylinder_entfernt_folge>"
  Bus Selector2/5 -> Add4/3  "<zylinder_entfernt_folge>"
  Add5/1 -> Data Type Conversion4/1
  Bus Selector/6 -> Add5/1  "<folge_belegt>"
  Bus Selector1/6 -> Add5/2  "<folge_belegt>"
  Bus Selector2/6 -> Add5/3  "<folge_belegt>"
  Add/1 -> Data Type Conversion/1
  Add1/1 -> Data Type Conversion1/1
  Data Type Conversion2/1 -> Bus Creator/4  "arbeitsraum_frei"
  Add4/1 -> Data Type Conversion3/1
  Data Type Conversion4/1 -> Bus Creator/6  "folge_belegt"

== system Vorlage_Anlagenteil_Pruefen_Gruppen12/Simulation Physik/Ausschussrutsche/Triggered Subsystem ==
  Trigger : TriggerPort  VariantControl=(inherit)
  Add : Sum
  Constant : Constant
  Memory : Memory  InheritSampleTime=on
  zyl_in_ausschuss : Outport
  wires:
  Constant/1 -> Add/1
  Memory/1 -> Add/2
  Add/1 -> zyl_in_ausschuss/1, Memory/1

== system Vorlage_Anlagenteil_Pruefen_Gruppen12/Systemtest Simulation1/1_schwarz_mit_Deckel/Signal Builder10 ==
  Demux : Demux  Tag=STV Demux  Outputs=8
      settings: DisplayOption=none
  FromWs : FromWorkspace  Tag=STV FromWs  VariableName=tuvar
      SigBuilderData=|
      | common.afterFinalStr = 'Extrapolate'
      | common.sampleTime = 0
      | dataSet.timeRange = [0 11]
      | dataSet.name = 'Group 1'
      | sbobj.Groups.Name = 'Group 1'
      | sbobj.Groups.Signals(1).Name = 'aufzug_abwaerts'
      | sbobj.Groups.Signals(1).XData = [0 6 6 10.5 10.5 11]
      | sbobj.Groups.Signals(1).YData = [0 0 1 1 0 0]
      | sbobj.Groups.Signals(2).Name = 'aufzug_aufwaerts'
      | sbobj.Groups.Signals(2).XData = [0 0.5 0.5 5 5 11]
      | sbobj.Groups.Signals(2).YData = [0 0 1 1 0 0]
      | sbobj.Groups.Signals(3).Name = 'zylinder_ausschieben'
      | sbobj.Groups.Signals(3).XData = [0 5.5 5.5 6.2 6.2 11]
      | sbobj.Groups.Signals(3).YData = [0 0 1 1 0 0]
      | sbobj.Groups.Signals(4).Name = 'luft_an'
      | sbobj.Groups.Signals(4).XData = [0 5.5 5.5 7.5 7.5 11]
      | sbobj.Groups.Signals(4).YData = [0 0 1 1 0 0]
      | sbobj.Groups.Signals(5).Name = 'Signal 5'
      | sbobj.Groups.Signals(5).XData = [0 11]
      | sbobj.Groups.Signals(5).YData = [0 0]
      | sbobj.Groups.Signals(6).Name = 'Signal 6'
      | sbobj.Groups.Signals(6).XData = [0 11]
      | sbobj.Groups.Signals(6).YData = [0 0]
      | sbobj.Groups.Signals(7).Name = 'Signal 7'
      | sbobj.Groups.Signals(7).XData = [0 11]
      | sbobj.Groups.Signals(7).YData = [0 0]
      | sbobj.Groups.Signals(8).Name = 'station_frei'
      | sbobj.Groups.Signals(8).XData = [0 0.1 0.1 11]
      | sbobj.Groups.Signals(8).YData = [1 1 0 0]
      | sbobj.Groups.TimeRange = [0 11]
  aufzug_abwaerts : Outport  Tag=STV Outport  VectorParamsAs1DForOutWhenUnconnected=off
  aufzug_aufwaerts : Outport  Tag=STV Outport  Port=2  VectorParamsAs1DForOutWhenUnconnected=off
  zylinder_ausschieben : Outport  Tag=STV Outport  Port=3  VectorParamsAs1DForOutWhenUnconnected=off
  luft_an : Outport  Tag=STV Outport  Port=4  VectorParamsAs1DForOutWhenUnconnected=off
  Signal 5 : Outport  Tag=STV Outport  Port=5  VectorParamsAs1DForOutWhenUnconnected=off
  Signal 6 : Outport  Tag=STV Outport  Port=6  VectorParamsAs1DForOutWhenUnconnected=off
  Signal 7 : Outport  Tag=STV Outport  Port=7  VectorParamsAs1DForOutWhenUnconnected=off
  station_frei : Outport  Tag=STV Outport  Port=8  VectorParamsAs1DForOutWhenUnconnected=off
  wires:
  Demux/1 -> aufzug_abwaerts/1
  FromWs/1 -> Demux/1
  Demux/2 -> aufzug_aufwaerts/1
  Demux/3 -> zylinder_ausschieben/1
  Demux/4 -> luft_an/1
  Demux/5 -> Signal 5/1
  Demux/6 -> Signal 6/1
  Demux/7 -> Signal 7/1
  Demux/8 -> station_frei/1

== system Vorlage_Anlagenteil_Pruefen_Gruppen12/Systemtest Simulation1/1_schwarz_mit_Deckel/Signal Builder4 ==
  Demux : Demux  Tag=STV Demux  Outputs=6
      settings: DisplayOption=none
  FromWs : FromWorkspace  Tag=STV FromWs  VariableName=tuvar
      SigBuilderData=|
      | common.afterFinalStr = 'Extrapolate'
      | common.sampleTime = 0
      | dataSet.timeRange = [0 11]
      | dataSet.name = 'Group 1'
      | sbobj.Groups.Name = 'Group 1'
      | sbobj.Groups.Signals(1).Name = 'zylinder_platziert'
      | sbobj.Groups.Signals(1).XData = [0 0.3 0.3 11]
      | sbobj.Groups.Signals(1).YData = [1 1 0 0]
      | sbobj.Groups.Signals(2).Name = 'zylinder_schwarz'
      | sbobj.Groups.Signals(2).XData = [0 5.6 5.6 11]
      | sbobj.Groups.Signals(2).YData = [1 1 0 0]
      | sbobj.Groups.Signals(3).Name = 'zylinder_hoehe'
      | sbobj.Groups.Signals(3).XData = [0 5 5 5.6 5.6 11]
      | sbobj.Groups.Signals(3).YData = [0 0 25 25 0 0]
      | sbobj.Groups.Signals(4).Name = 'arbeitsraum_frei'
      | sbobj.Groups.Signals(4).XData = [0 0.5 0.5 10.5 10.5 10.8 10.8 11]
      | sbobj.Groups.Signals(4).YData = [1 1 0 0 1 1 0 0]
      | sbobj.Groups.Signals(5).Name = 'zylinder_entfernt_folge'
      | sbobj.Groups.Signals(5).XData = [0 10 10 10.5 10.5 11]
      | sbobj.Groups.Signals(5).YData = [0 0 1 1 0 0]
      | sbobj.Groups.Signals(6).Name = 'folge_belegt'
      | sbobj.Groups.Signals(6).XData = [0 4 4 5.5 5.5 11]
      | sbobj.Groups.Signals(6).YData = [0 0 1 1 0 0]
      | sbobj.Groups.TimeRange = [0 11]
  zylinder_platziert : Outport  Tag=STV Outport  VectorParamsAs1DForOutWhenUnconnected=off
  zylinder_schwarz : Outport  Tag=STV Outport  Port=2  VectorParamsAs1DForOutWhenUnconnected=off
  zylinder_hoehe : Outport  Tag=STV Outport  Port=3  VectorParamsAs1DForOutWhenUnconnected=off
  arbeitsraum_frei : Outport  Tag=STV Outport  Port=4  VectorParamsAs1DForOutWhenUnconnected=off
  zylinder_entfernt_folge : Outport  Tag=STV Outport  Port=5  VectorParamsAs1DForOutWhenUnconnected=off
  folge_belegt : Outport  Tag=STV Outport  Port=6  VectorParamsAs1DForOutWhenUnconnected=off
  wires:
  Demux/1 -> zylinder_platziert/1
  FromWs/1 -> Demux/1
  Demux/2 -> zylinder_schwarz/1
  Demux/3 -> zylinder_hoehe/1
  Demux/4 -> arbeitsraum_frei/1
  Demux/5 -> zylinder_entfernt_folge/1
  Demux/6 -> folge_belegt/1

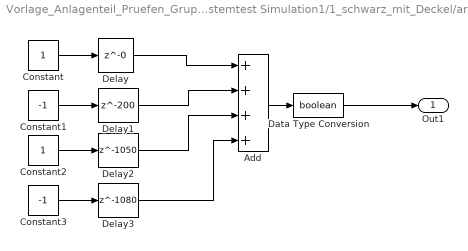
== system Vorlage_Anlagenteil_Pruefen_Gruppen12/Systemtest Simulation1/1_schwarz_mit_Deckel/arbeitsraum_frei ==
  Add : Sum  Inputs=++++
  Constant : Constant
  Constant1 : Constant  Value=-1
  Constant2 : Constant
  Constant3 : Constant  Value=-1
  Data Type Conversion : DataTypeConversion  OutDataTypeStr=boolean  SaturateOnIntegerOverflow=off  RndMeth=Floor
  Delay : Delay  DelayLength=0
  Delay1 : Delay  DelayLength=200
  Delay2 : Delay  DelayLength=1050
  Delay3 : Delay  DelayLength=1080
  Out1 : Outport  VectorParamsAs1DForOutWhenUnconnected=off
  wires:
  Constant/1 -> Delay/1
  Constant1/1 -> Delay1/1
  Delay/1 -> Add/1
  Delay1/1 -> Add/2
  Add/1 -> Data Type Conversion/1
  Data Type Conversion/1 -> Out1/1
  Constant2/1 -> Delay2/1
  Delay2/1 -> Add/3
  Constant3/1 -> Delay3/1
  Delay3/1 -> Add/4

== system Vorlage_Anlagenteil_Pruefen_Gruppen12/Systemtest Simulation1/1_schwarz_mit_Deckel/aufzug_abwaerts ==
  Add : Sum
  Constant : Constant
  Constant1 : Constant  Value=-1
  Data Type Conversion : DataTypeConversion  OutDataTypeStr=boolean  SaturateOnIntegerOverflow=off  RndMeth=Floor
  Delay : Delay  DelayLength=600
  Delay1 : Delay  DelayLength=1050
  Out1 : Outport  VectorParamsAs1DForOutWhenUnconnected=off
  wires:
  Constant/1 -> Delay/1
  Constant1/1 -> Delay1/1
  Delay/1 -> Add/1
  Delay1/1 -> Add/2
  Add/1 -> Data Type Conversion/1
  Data Type Conversion/1 -> Out1/1

== system Vorlage_Anlagenteil_Pruefen_Gruppen12/Systemtest Simulation1/1_schwarz_mit_Deckel/aufzug_aufwaerts ==
  Add : Sum
  Constant : Constant
  Constant1 : Constant  Value=-1
  Data Type Conversion : DataTypeConversion  OutDataTypeStr=boolean  SaturateOnIntegerOverflow=off  RndMeth=Floor
  Delay : Delay  DelayLength=50
  Delay1 : Delay  DelayLength=500
  Out1 : Outport  VectorParamsAs1DForOutWhenUnconnected=off
  wires:
  Constant/1 -> Delay/1
  Constant1/1 -> Delay1/1
  Delay/1 -> Add/1
  Delay1/1 -> Add/2
  Add/1 -> Data Type Conversion/1
  Data Type Conversion/1 -> Out1/1

== system Vorlage_Anlagenteil_Pruefen_Gruppen12/Systemtest Simulation1/1_schwarz_mit_Deckel/done_signal ==
  Constant : Constant
  Data Type Conversion : DataTypeConversion  OutDataTypeStr=boolean  SaturateOnIntegerOverflow=off  RndMeth=Floor
  Delay : Delay  DelayLength=1080
  Out1 : Outport  VectorParamsAs1DForOutWhenUnconnected=off
  wires:
  Constant/1 -> Delay/1
  Data Type Conversion/1 -> Out1/1
  Delay/1 -> Data Type Conversion/1

== system Vorlage_Anlagenteil_Pruefen_Gruppen12/Systemtest Simulation1/1_schwarz_mit_Deckel/folge_belegt ==
  Add : Sum
  Constant1 : Constant
  Constant2 : Constant  Value=-1
  Data Type Conversion1 : DataTypeConversion  OutDataTypeStr=boolean  SaturateOnIntegerOverflow=off  RndMeth=Floor
  Delay : Delay  DelayLength=400
  Delay1 : Delay  DelayLength=550
  Out1 : Outport  VectorParamsAs1DForOutWhenUnconnected=off
  wires:
  Data Type Conversion1/1 -> Out1/1
  Constant1/1 -> Delay/1
  Constant2/1 -> Delay1/1
  Delay/1 -> Add/1
  Delay1/1 -> Add/2
  Add/1 -> Data Type Conversion1/1

== system Vorlage_Anlagenteil_Pruefen_Gruppen12/Systemtest Simulation1/1_schwarz_mit_Deckel/luft_an ==
  Add : Sum
  Constant : Constant
  Constant1 : Constant  Value=-1
  Data Type Conversion : DataTypeConversion  OutDataTypeStr=boolean  SaturateOnIntegerOverflow=off  RndMeth=Floor
  Delay : Delay  DelayLength=550
  Delay1 : Delay  DelayLength=750
  Out1 : Outport  VectorParamsAs1DForOutWhenUnconnected=off
  wires:
  Constant/1 -> Delay/1
  Constant1/1 -> Delay1/1
  Delay/1 -> Add/1
  Delay1/1 -> Add/2
  Add/1 -> Data Type Conversion/1
  Data Type Conversion/1 -> Out1/1

== system Vorlage_Anlagenteil_Pruefen_Gruppen12/Systemtest Simulation1/1_schwarz_mit_Deckel/out5 ==
  Add : Sum
  Constant : Constant
  Constant1 : Constant  Value=-1
  Data Type Conversion : DataTypeConversion  OutDataTypeStr=boolean  SaturateOnIntegerOverflow=off  RndMeth=Floor
  Delay : Delay  DelayLength=0
  Delay1 : Delay  DelayLength=0
  Out1 : Outport  VectorParamsAs1DForOutWhenUnconnected=off
  wires:
  Constant/1 -> Delay/1
  Constant1/1 -> Delay1/1
  Delay/1 -> Add/1
  Delay1/1 -> Add/2
  Add/1 -> Data Type Conversion/1
  Data Type Conversion/1 -> Out1/1

== system Vorlage_Anlagenteil_Pruefen_Gruppen12/Systemtest Simulation1/1_schwarz_mit_Deckel/out6 ==
  Add : Sum
  Constant : Constant
  Constant1 : Constant  Value=-1
  Data Type Conversion : DataTypeConversion  OutDataTypeStr=boolean  SaturateOnIntegerOverflow=off  RndMeth=Floor
  Delay : Delay  DelayLength=0
  Delay1 : Delay  DelayLength=0
  Out1 : Outport  VectorParamsAs1DForOutWhenUnconnected=off
  wires:
  Constant/1 -> Delay/1
  Constant1/1 -> Delay1/1
  Delay/1 -> Add/1
  Delay1/1 -> Add/2
  Add/1 -> Data Type Conversion/1
  Data Type Conversion/1 -> Out1/1

== system Vorlage_Anlagenteil_Pruefen_Gruppen12/Systemtest Simulation1/1_schwarz_mit_Deckel/out7 ==
  Add : Sum
  Constant : Constant
  Constant1 : Constant  Value=-1
  Data Type Conversion : DataTypeConversion  OutDataTypeStr=boolean  SaturateOnIntegerOverflow=off  RndMeth=Floor
  Delay : Delay  DelayLength=0
  Delay1 : Delay  DelayLength=0
  Out1 : Outport  VectorParamsAs1DForOutWhenUnconnected=off
  wires:
  Constant/1 -> Delay/1
  Constant1/1 -> Delay1/1
  Delay/1 -> Add/1
  Delay1/1 -> Add/2
  Add/1 -> Data Type Conversion/1
  Data Type Conversion/1 -> Out1/1

== system Vorlage_Anlagenteil_Pruefen_Gruppen12/Systemtest Simulation1/1_schwarz_mit_Deckel/station_frei ==
  Add : Sum
  Constant : Constant
  Constant1 : Constant  Value=-1
  Data Type Conversion : DataTypeConversion  OutDataTypeStr=boolean  SaturateOnIntegerOverflow=off  RndMeth=Floor
  Delay : Delay  DelayLength=0
  Delay1 : Delay  DelayLength=10
  Out1 : Outport  VectorParamsAs1DForOutWhenUnconnected=off
  wires:
  Constant/1 -> Delay/1
  Constant1/1 -> Delay1/1
  Delay/1 -> Add/1
  Delay1/1 -> Add/2
  Add/1 -> Data Type Conversion/1
  Data Type Conversion/1 -> Out1/1

== system Vorlage_Anlagenteil_Pruefen_Gruppen12/Systemtest Simulation1/1_schwarz_mit_Deckel/zylinder_ausschieben ==
  Add : Sum
  Constant : Constant
  Constant1 : Constant  Value=-1
  Data Type Conversion : DataTypeConversion  OutDataTypeStr=boolean  SaturateOnIntegerOverflow=off  RndMeth=Floor
  Delay : Delay  DelayLength=550
  Delay1 : Delay  DelayLength=620
  Out1 : Outport  VectorParamsAs1DForOutWhenUnconnected=off
  wires:
  Constant/1 -> Delay/1
  Constant1/1 -> Delay1/1
  Delay/1 -> Add/1
  Delay1/1 -> Add/2
  Add/1 -> Data Type Conversion/1
  Data Type Conversion/1 -> Out1/1

== system Vorlage_Anlagenteil_Pruefen_Gruppen12/Systemtest Simulation1/1_schwarz_mit_Deckel/zylinder_entfernt_folge ==
  Add : Sum
  Constant : Constant
  Constant1 : Constant  Value=-1
  Data Type Conversion : DataTypeConversion  OutDataTypeStr=boolean  SaturateOnIntegerOverflow=off  RndMeth=Floor
  Delay : Delay  DelayLength=1000
  Delay1 : Delay  DelayLength=1050
  Out1 : Outport  VectorParamsAs1DForOutWhenUnconnected=off
  wires:
  Constant/1 -> Delay/1
  Constant1/1 -> Delay1/1
  Delay/1 -> Add/1
  Delay1/1 -> Add/2
  Add/1 -> Data Type Conversion/1
  Data Type Conversion/1 -> Out1/1

== system Vorlage_Anlagenteil_Pruefen_Gruppen12/Systemtest Simulation1/1_schwarz_mit_Deckel/zylinder_hoehe ==
  Add : Sum
  Constant : Constant  Value=25
  Constant1 : Constant  Value=-25
  Delay : Delay  DelayLength=50
  Delay1 : Delay  DelayLength=900
  Out1 : Outport  VectorParamsAs1DForOutWhenUnconnected=off
  wires:
  Constant/1 -> Delay/1
  Constant1/1 -> Delay1/1
  Delay/1 -> Add/1
  Delay1/1 -> Add/2
  Add/1 -> Out1/1

== system Vorlage_Anlagenteil_Pruefen_Gruppen12/Systemtest Simulation1/1_schwarz_mit_Deckel/zylinder_platziert ==
  Add : Sum
  Constant : Constant
  Constant1 : Constant  Value=-1
  Data Type Conversion : DataTypeConversion  OutDataTypeStr=boolean  SaturateOnIntegerOverflow=off  RndMeth=Floor
  Delay : Delay  DelayLength=50
  Delay1 : Delay  DelayLength=70
  Out1 : Outport  VectorParamsAs1DForOutWhenUnconnected=off
  wires:
  Constant/1 -> Delay/1
  Constant1/1 -> Delay1/1
  Delay/1 -> Add/1
  Delay1/1 -> Add/2
  Add/1 -> Data Type Conversion/1
  Data Type Conversion/1 -> Out1/1

== system Vorlage_Anlagenteil_Pruefen_Gruppen12/Systemtest Simulation1/1_schwarz_mit_Deckel/zylinder_schwarz ==
  Add : Sum
  Constant : Constant
  Constant1 : Constant  Value=-1
  Data Type Conversion : DataTypeConversion  OutDataTypeStr=boolean  SaturateOnIntegerOverflow=off  RndMeth=Floor
  Delay : Delay  DelayLength=0
  Delay1 : Delay  DelayLength=700
  Out1 : Outport  VectorParamsAs1DForOutWhenUnconnected=off
  wires:
  Constant/1 -> Delay/1
  Constant1/1 -> Delay1/1
  Delay/1 -> Add/1
  Delay1/1 -> Add/2
  Add/1 -> Data Type Conversion/1
  Data Type Conversion/1 -> Out1/1

== system Vorlage_Anlagenteil_Pruefen_Gruppen12/Systemtest Simulation1/2_rot_mit_Deckel/Signal Builder10 ==
  Demux : Demux  Tag=STV Demux  Outputs=8
      settings: DisplayOption=none
  FromWs : FromWorkspace  Tag=STV FromWs  VariableName=tuvar
      SigBuilderData=|
      | common.afterFinalStr = 'Extrapolate'
      | common.sampleTime = 0
      | dataSet.timeRange = [0 11]
      | dataSet.name = 'Group 1'
      | sbobj.Groups.Name = 'Group 1'
      | sbobj.Groups.Signals(1).Name = 'aufzug_abwaerts'
      | sbobj.Groups.Signals(1).XData = [0 6 6 10.5 10.5 11]
      | sbobj.Groups.Signals(1).YData = [0 0 1 1 0 0]
      | sbobj.Groups.Signals(2).Name = 'aufzug_aufwaerts'
      | sbobj.Groups.Signals(2).XData = [0 0.5 0.5 5 5 11]
      | sbobj.Groups.Signals(2).YData = [0 0 1 1 0 0]
      | sbobj.Groups.Signals(3).Name = 'zylinder_ausschieben'
      | sbobj.Groups.Signals(3).XData = [0 5.5 5.5 6.2 6.2 11]
      | sbobj.Groups.Signals(3).YData = [0 0 1 1 0 0]
      | sbobj.Groups.Signals(4).Name = 'luft_an'
      | sbobj.Groups.Signals(4).XData = [0 5.5 5.5 7.5 7.5 11]
      | sbobj.Groups.Signals(4).YData = [0 0 1 1 0 0]
      | sbobj.Groups.Signals(5).Name = 'Signal 5'
      | sbobj.Groups.Signals(5).XData = [0 11]
      | sbobj.Groups.Signals(5).YData = [0 0]
      | sbobj.Groups.Signals(6).Name = 'Signal 6'
      | sbobj.Groups.Signals(6).XData = [0 11]
      | sbobj.Groups.Signals(6).YData = [0 0]
      | sbobj.Groups.Signals(7).Name = 'Signal 7'
      | sbobj.Groups.Signals(7).XData = [0 11]
      | sbobj.Groups.Signals(7).YData = [0 0]
      | sbobj.Groups.Signals(8).Name = 'station_frei'
      | sbobj.Groups.Signals(8).XData = [0 0.1 0.1 11]
      | sbobj.Groups.Signals(8).YData = [1 1 0 0]
      | sbobj.Groups.TimeRange = [0 11]
  aufzug_abwaerts : Outport  Tag=STV Outport  VectorParamsAs1DForOutWhenUnconnected=off
  aufzug_aufwaerts : Outport  Tag=STV Outport  Port=2  VectorParamsAs1DForOutWhenUnconnected=off
  zylinder_ausschieben : Outport  Tag=STV Outport  Port=3  VectorParamsAs1DForOutWhenUnconnected=off
  luft_an : Outport  Tag=STV Outport  Port=4  VectorParamsAs1DForOutWhenUnconnected=off
  Signal 5 : Outport  Tag=STV Outport  Port=5  VectorParamsAs1DForOutWhenUnconnected=off
  Signal 6 : Outport  Tag=STV Outport  Port=6  VectorParamsAs1DForOutWhenUnconnected=off
  Signal 7 : Outport  Tag=STV Outport  Port=7  VectorParamsAs1DForOutWhenUnconnected=off
  station_frei : Outport  Tag=STV Outport  Port=8  VectorParamsAs1DForOutWhenUnconnected=off
  wires:
  Demux/1 -> aufzug_abwaerts/1
  FromWs/1 -> Demux/1
  Demux/2 -> aufzug_aufwaerts/1
  Demux/3 -> zylinder_ausschieben/1
  Demux/4 -> luft_an/1
  Demux/5 -> Signal 5/1
  Demux/6 -> Signal 6/1
  Demux/7 -> Signal 7/1
  Demux/8 -> station_frei/1

== system Vorlage_Anlagenteil_Pruefen_Gruppen12/Systemtest Simulation1/2_rot_mit_Deckel/Signal Builder4 ==
  Demux : Demux  Tag=STV Demux  Outputs=6
      settings: DisplayOption=none
  FromWs : FromWorkspace  Tag=STV FromWs  VariableName=tuvar
      SigBuilderData=|
      | common.afterFinalStr = 'Extrapolate'
      | common.sampleTime = 0
      | dataSet.timeRange = [0 11]
      | dataSet.name = 'Group 1'
      | sbobj.Groups.Name = 'Group 1'
      | sbobj.Groups.Signals(1).Name = 'zylinder_platziert'
      | sbobj.Groups.Signals(1).XData = [0 0.3 0.3 11]
      | sbobj.Groups.Signals(1).YData = [1 1 0 0]
      | sbobj.Groups.Signals(2).Name = 'zylinder_schwarz'
      | sbobj.Groups.Signals(2).XData = [0 11]
      | sbobj.Groups.Signals(2).YData = [0 0]
      | sbobj.Groups.Signals(3).Name = 'zylinder_hoehe'
      | sbobj.Groups.Signals(3).XData = [0 5 5 5.6 5.6 11]
      | sbobj.Groups.Signals(3).YData = [0 0 28 28 0 0]
      | sbobj.Groups.Signals(4).Name = 'arbeitsraum_frei'
      | sbobj.Groups.Signals(4).XData = [0 0.5 0.5 10.5 10.5 10.8 10.8 11]
      | sbobj.Groups.Signals(4).YData = [1 1 0 0 1 1 0 0]
      | sbobj.Groups.Signals(5).Name = 'zylinder_entfernt_folge'
      | sbobj.Groups.Signals(5).XData = [0 10 10 10.5 10.5 11]
      | sbobj.Groups.Signals(5).YData = [0 0 1 1 0 0]
      | sbobj.Groups.Signals(6).Name = 'folge_belegt'
      | sbobj.Groups.Signals(6).XData = [0 4 5.5 11]
      | sbobj.Groups.Signals(6).YData = [0 0 0 0]
      | sbobj.Groups.TimeRange = [0 11]
  zylinder_platziert : Outport  Tag=STV Outport  VectorParamsAs1DForOutWhenUnconnected=off
  zylinder_schwarz : Outport  Tag=STV Outport  Port=2  VectorParamsAs1DForOutWhenUnconnected=off
  zylinder_hoehe : Outport  Tag=STV Outport  Port=3  VectorParamsAs1DForOutWhenUnconnected=off
  arbeitsraum_frei : Outport  Tag=STV Outport  Port=4  VectorParamsAs1DForOutWhenUnconnected=off
  zylinder_entfernt_folge : Outport  Tag=STV Outport  Port=5  VectorParamsAs1DForOutWhenUnconnected=off
  folge_belegt : Outport  Tag=STV Outport  Port=6  VectorParamsAs1DForOutWhenUnconnected=off
  wires:
  Demux/1 -> zylinder_platziert/1
  FromWs/1 -> Demux/1
  Demux/2 -> zylinder_schwarz/1
  Demux/3 -> zylinder_hoehe/1
  Demux/4 -> arbeitsraum_frei/1
  Demux/5 -> zylinder_entfernt_folge/1
  Demux/6 -> folge_belegt/1

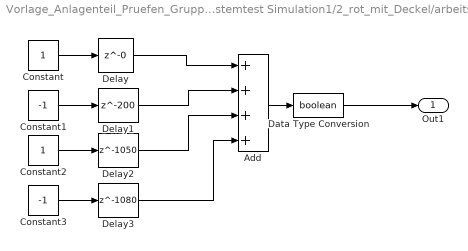
== system Vorlage_Anlagenteil_Pruefen_Gruppen12/Systemtest Simulation1/2_rot_mit_Deckel/arbeitsraum_frei ==
  Add : Sum  Inputs=++++
  Constant : Constant
  Constant1 : Constant  Value=-1
  Constant2 : Constant
  Constant3 : Constant  Value=-1
  Data Type Conversion : DataTypeConversion  OutDataTypeStr=boolean  SaturateOnIntegerOverflow=off  RndMeth=Floor
  Delay : Delay  DelayLength=0
  Delay1 : Delay  DelayLength=200
  Delay2 : Delay  DelayLength=1050
  Delay3 : Delay  DelayLength=1080
  Out1 : Outport  VectorParamsAs1DForOutWhenUnconnected=off
  wires:
  Constant/1 -> Delay/1
  Constant1/1 -> Delay1/1
  Delay/1 -> Add/1
  Delay1/1 -> Add/2
  Add/1 -> Data Type Conversion/1
  Data Type Conversion/1 -> Out1/1
  Constant2/1 -> Delay2/1
  Delay2/1 -> Add/3
  Constant3/1 -> Delay3/1
  Delay3/1 -> Add/4

== system Vorlage_Anlagenteil_Pruefen_Gruppen12/Systemtest Simulation1/2_rot_mit_Deckel/aufzug_abwaerts ==
  Add : Sum
  Constant : Constant
  Constant1 : Constant  Value=-1
  Data Type Conversion : DataTypeConversion  OutDataTypeStr=boolean  SaturateOnIntegerOverflow=off  RndMeth=Floor
  Delay : Delay  DelayLength=600
  Delay1 : Delay  DelayLength=1050
  Out1 : Outport  VectorParamsAs1DForOutWhenUnconnected=off
  wires:
  Constant/1 -> Delay/1
  Constant1/1 -> Delay1/1
  Delay/1 -> Add/1
  Delay1/1 -> Add/2
  Add/1 -> Data Type Conversion/1
  Data Type Conversion/1 -> Out1/1

== system Vorlage_Anlagenteil_Pruefen_Gruppen12/Systemtest Simulation1/2_rot_mit_Deckel/aufzug_aufwaerts ==
  Add : Sum
  Constant : Constant
  Constant1 : Constant  Value=-1
  Data Type Conversion : DataTypeConversion  OutDataTypeStr=boolean  SaturateOnIntegerOverflow=off  RndMeth=Floor
  Delay : Delay  DelayLength=50
  Delay1 : Delay  DelayLength=500
  Out1 : Outport  VectorParamsAs1DForOutWhenUnconnected=off
  wires:
  Constant/1 -> Delay/1
  Constant1/1 -> Delay1/1
  Delay/1 -> Add/1
  Delay1/1 -> Add/2
  Add/1 -> Data Type Conversion/1
  Data Type Conversion/1 -> Out1/1

== system Vorlage_Anlagenteil_Pruefen_Gruppen12/Systemtest Simulation1/2_rot_mit_Deckel/done_signal ==
  Constant : Constant
  Data Type Conversion : DataTypeConversion  OutDataTypeStr=boolean  SaturateOnIntegerOverflow=off  RndMeth=Floor
  Delay : Delay  DelayLength=1080
  Out1 : Outport  VectorParamsAs1DForOutWhenUnconnected=off
  wires:
  Constant/1 -> Delay/1
  Data Type Conversion/1 -> Out1/1
  Delay/1 -> Data Type Conversion/1
